simulink model "DC_motor"  (R2022b)
settings: Solver=VariableStepAuto  StartTime=0.0  StopTime=0.2  RelTol=1e-3
values from neighbouring files (symbols this model uses):
  b = 5.8/6*1e-4    (= 9.66666666667e-05)    [DC_motor_mfile.m]
  D_adm = 2*zeta_adm*wn_adm*M_adm    (= 20)    [DC_motor_mfile.m]    (also in oneDim_mfile.m = 1)
  g = 9.807    [DC_motor_mfile.m]    (also in oneDim_mfile.m)
  J = 5.8e-7    (= 5.8e-07)    [DC_motor_mfile.m]
  K_adm = wn_adm^2*M_adm    (= 100)    [DC_motor_mfile.m]    (also in oneDim_mfile.m = 2.5)
  K_D_pos = (2*zeta_m_pos*wn_m_pos*T - 1)/K    (= 0.0265230129141)    [DC_motor_mfile.m]
  K_D_pos_pass = 2*zeta_m_pos*wn_m_pos    (= 200)    [DC_motor_mfile.m]
  K_I_pos = 0    [DC_motor_mfile.m]
  K_P_pos = wn_m_pos^2 * T/K    (= 9.86111111111)    [DC_motor_mfile.m]
  K_P_pos_pass = wn_m_pos^2    (= 10000)    [DC_motor_mfile.m]
  Kb = 2.73e-3*(60/(2*pi))    (= 0.0260695796785)    [DC_motor_mfile.m]
  Km = 26.1e-3    (= 0.0261)    [DC_motor_mfile.m]
  L = 1    [DC_motor_mfile.m]
  m = 1    [DC_motor_mfile.m]    (also in oneDim_mfile.m = 0.5)
  M_adm = 1    [DC_motor_mfile.m]    (also in oneDim_mfile.m = 0.1)
  Ra = 7.1    [DC_motor_mfile.m]
  simpDC_gain = Km/(Ra*b+Kb*Km)    (= 19.0964054623)    [DC_motor_mfile.m]
  simpDC_timeconst = (Ra*J/(Ra*b+Kb*Km))    (= 0.00301298841738)    [DC_motor_mfile.m]
libraries: lib_robot x20
settings Model: Creator=chris  LastModifiedBy=chris

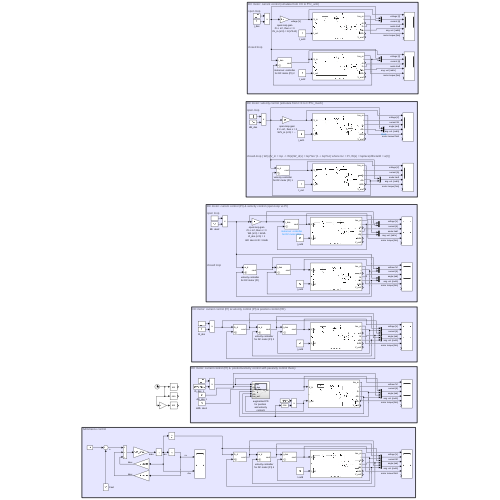
[thumbnail: Simulink's stored preview of the top-level diagram]
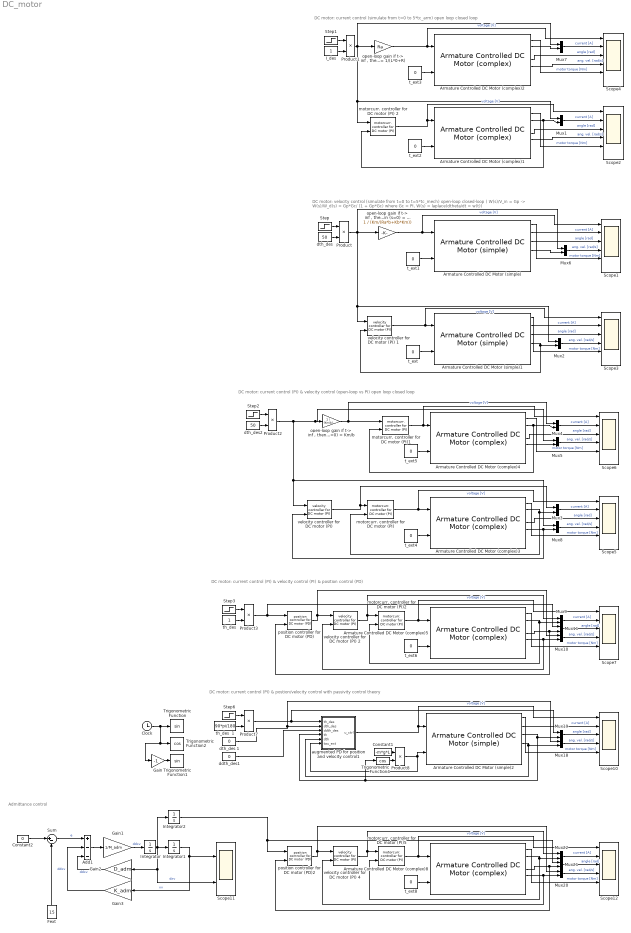
== system DC_motor ==
  note: Admittance control
  note: DC motor: current control (PI) & velocity control (PI) & position control (PD)
  note: DC motor: current control (PI) & velocity control (open-loop vs PI)
      |
      | open loop
      |
      |
      |
      |
      |
      |
      |
      |
      |
      |
      |
      |
      |
      |
      |
      | closed loop
  note: DC motor: current control (simulate from t=0 to 5*tc_arm)
      |
      | open loop
      |
      |
      |
      |
      |
      |
      |
      |
      |
      |
      | closed loop
  note: DC motor: velocity control (simulate from t=0 to t=5*tc_mech)
      |
      | open-loop
      |
      |
      |
      |
      |
      |
      |
      |
      |
      |
      |
      |
      |
      | closed-loop ( W(s)/V_in = Gp -> W(s)/W_d(s) = Gp*Gc/ (1 + Gp*Gc) where Gc = PI, W(s) = laplace(dtheta/dt = w(t))
  note: DC motor: current control (PI) & postion/velocity control with passivity control theory
  Add1 : Sum  Inputs=+--
  Armature Controlled DC Motor (complex){1..5,8} (6 alike) : lib_robot/Armature Controlled DC Motor (complex)  SystemSampleTime=-1  VariantActivationTime=update diagram  Latency=0  AutoFrameSizeCalculation=off
  Armature Controlled DC Motor (simple) : lib_robot/Armature Controlled DC Motor (simple)  SystemSampleTime=-1  VariantActivationTime=update diagram  Latency=0  AutoFrameSizeCalculation=off
  Armature Controlled DC Motor (simple)1 : lib_robot/Armature Controlled DC Motor (simple)  SystemSampleTime=-1  VariantActivationTime=update diagram  Latency=0  AutoFrameSizeCalculation=off
  Armature Controlled DC Motor (simple)2 : lib_robot/Armature Controlled DC Motor (simple)  SystemSampleTime=-1  VariantActivationTime=update diagram  Latency=0  AutoFrameSizeCalculation=off
  Clock : Clock
  Constant1 : Constant  Value=-m*g*L
  Constant2 : Constant  Value=0
  Fext : Constant  Value=15
  Gain : Gain  Gain=-1
  Gain1 : Gain  Gain=1/M_adm
  Gain2 : Gain  Gain=D_adm
  Gain3 : Gain  Gain=K_adm
  I_des : Constant
  Integrator : Integrator
  Integrator1 : Integrator
  Integrator2 : Integrator
  Mux{1..11,18..22} (16 alike) : Mux  Inputs=2
  Product{,1..3,7..8} (6 alike) : Product
  Scope{1..7,10,12} (9 alike) : Scope  NumInputPorts=6
  Scope11 : Scope  NumInputPorts=2
  Step{,1..3} (4 alike) : Step  Time=0  SampleTime=0
  Step6 : Step  Time=0.1  SampleTime=0
  Sum : Sum  Inputs=|+-
  Trigonometric Function : Trigonometry
  Trigonometric Function1 : Trigonometry
  Trigonometric Function2 : Trigonometry  Operator=cos
  Trigonometric Function4 : Trigonometry  Operator=cos
  augmented PD for position and velocity control1 : Subsystem
  ddth_des1 : Constant  Value=0
  dth_des : Constant  Value=50
  dth_des 1 : Constant  Value=0
  dth_des2 : Constant  Value=50
  motorcurr. controller for DC motor (PI){,1..2,5} (4 alike) : lib_robot/motorcurr. controller for DC motor (PI)  mask_K_P=K_P_cur  mask_K_I=K_I_cur
  motorcurr. controller for DC motor (PI) 2 : lib_robot/motorcurr. controller for DC motor (PI)  mask_K_P=K_P_cur  mask_K_I=K_I_cur
  "open-loop gain if t-> inf , then s = 0 I/V_in (s=0) = 1/(L*0+R)" : Gain  Gain=Ra
  "open-loop gain if t-> inf , then s = 0 W/I (s=0) = Km/b I/I_des (s=0) = 1 W/I_des (s=0) = Km/b" : Gain  Gain=1 / (Km/b)
  "open-loop gain if t-> inf , then s = 0 W/V_in (s=0) = ... " : Gain  Gain=1 / (Km/(Ra*b+Kb*Km))
  position controller for DC motor (PD) : lib_robot/position controller for DC motor (PD)  P=K_P_pos  I=K_I_pos  D=K_D_pos  N=100
  position controller for DC motor (PD)2 : lib_robot/position controller for DC motor (PD)  P=K_P_pos  I=K_I_pos  D=K_D_pos  N=100
  t_ext{,1..6,8} (8 alike) : Constant  Value=0
  th_des : Constant
  th_des  1 : Constant  Value=90*pi/180
  velocity controller for DC motor (PI) {,1..2,4} (4 alike) : lib_robot/velocity controller for DC motor (PI)  mask_K_P=K_P_vel  mask_K_I=K_I_vel
  wires:
  t_ext/1 -> Armature Controlled DC Motor (simple)1/2
  Product/1 -> "open-loop gain if t-> inf , then s = 0 W/V_in (s=0) = ... "/1, Mux6/1, velocity controller for DC motor (PI) 1/1, Mux2/1
  Armature Controlled DC Motor (simple)1/3 -> Scope3/3  "angle [rad]"
  Armature Controlled DC Motor (simple)1/4 -> velocity controller for DC motor (PI) 1/2, Mux2/2
  velocity controller for DC motor (PI) 1/1 -> Scope3/1, Armature Controlled DC Motor (simple)1/1  "voltage [V]"
  Armature Controlled DC Motor (simple)1/2 -> Scope3/2  "current [A]"
  Mux2/1 -> Scope3/4  "ang. vel. [rad/s]"
  Armature Controlled DC Motor (simple)1/1 -> Scope3/5  "motor torque [Nm]"
  t_ext1/1 -> Armature Controlled DC Motor (simple)/2
  Armature Controlled DC Motor (simple)/3 -> Scope1/3  "angle [rad]"
  Armature Controlled DC Motor (simple)/1 -> Scope1/5  "motor torque [Nm]"
  Mux6/1 -> Scope1/4  "ang. vel. [rad/s]"
  "open-loop gain if t-> inf , then s = 0 W/V_in (s=0) = ... "/1 -> Scope1/1, Armature Controlled DC Motor (simple)/1  "voltage [V]"
  Armature Controlled DC Motor (simple)/2 -> Scope1/2  "current [A]"
  Step/1 -> Product/1
  dth_des/1 -> Product/2
  Armature Controlled DC Motor (complex)1/4 -> Scope2/3  "angle [rad]"
  Armature Controlled DC Motor (complex)1/1 -> Scope2/5  "motor torque [Nm]"
  Armature Controlled DC Motor (complex)1/2 -> motorcurr. controller for DC motor (PI) 2/2, Mux1/2
  t_ext2/1 -> Armature Controlled DC Motor (complex)1/2
  Product1/1 -> "open-loop gain if t-> inf , then s = 0 I/V_in (s=0) = 1/(L*0+R)"/1, Mux7/1, motorcurr. controller for DC motor (PI) 2/1, Mux1/1
  Armature Controlled DC Motor (complex)1/5 -> Scope2/4  "ang. vel. [rad/s]"
  motorcurr. controller for DC motor (PI) 2/1 -> Scope2/1, Armature Controlled DC Motor (complex)1/1  "voltage [V]"
  Mux1/1 -> Scope2/2  "current [A]"
  t_ext3/1 -> Armature Controlled DC Motor (complex)2/2
  Armature Controlled DC Motor (complex)2/1 -> Scope4/5  "motor torque [Nm]"
  Mux7/1 -> Scope4/2  "current [A]"
  Armature Controlled DC Motor (complex)2/4 -> Scope4/3  "angle [rad]"
  "open-loop gain if t-> inf , then s = 0 I/V_in (s=0) = 1/(L*0+R)"/1 -> Scope4/1, Armature Controlled DC Motor (complex)2/1  "voltage [V]"
  Armature Controlled DC Motor (complex)2/5 -> Scope4/4  "ang. vel. [rad/s]"
  t_ext4/1 -> Armature Controlled DC Motor (complex)3/2
  Armature Controlled DC Motor (complex)3/5 -> "velocity controller for DC motor (PI) "/2, Mux8/2
  Product2/1 -> "velocity controller for DC motor (PI) "/1, Mux8/1, Mux5/1, "open-loop gain if t-> inf , then s = 0 W/I (s=0) = Km/b I/I_des (s=0) = 1 W/I_des (s=0) = Km/b"/1
  t_ext5/1 -> Armature Controlled DC Motor (complex)4/2
  Mux5/1 -> Scope6/4  "ang. vel. [rad/s]"
  Armature Controlled DC Motor (complex)4/1 -> Scope6/5  "motor torque [Nm]"
  motorcurr. controller for DC motor (PI)1/1 -> Scope6/1, Armature Controlled DC Motor (complex)4/1  "voltage [V]"
  Armature Controlled DC Motor (complex)4/4 -> Scope6/3  "angle [rad]"
  Mux4/1 -> Scope6/2  "current [A]"
  Armature Controlled DC Motor (complex)4/2 -> motorcurr. controller for DC motor (PI)1/2, Mux4/2
  "open-loop gain if t-> inf , then s = 0 W/I (s=0) = Km/b I/I_des (s=0) = 1 W/I_des (s=0) = Km/b"/1 -> motorcurr. controller for DC motor (PI)1/1, Mux4/1
  Armature Controlled DC Motor (simple)/4 -> Mux6/2
  Armature Controlled DC Motor (complex)2/2 -> Mux7/2
  Armature Controlled DC Motor (complex)4/5 -> Mux5/2
  Mux3/1 -> Scope5/2  "current [A]"
  Mux8/1 -> Scope5/4  "ang. vel. [rad/s]"
  Armature Controlled DC Motor (complex)3/2 -> motorcurr. controller for DC motor (PI)/2, Mux3/2
  Armature Controlled DC Motor (complex)3/4 -> Scope5/3  "angle [rad]"
  Armature Controlled DC Motor (complex)3/1 -> Scope5/5  "motor torque [Nm]"
  "velocity controller for DC motor (PI) "/1 -> motorcurr. controller for DC motor (PI)/1, Mux3/1
  motorcurr. controller for DC motor (PI)/1 -> Armature Controlled DC Motor (complex)3/1, Scope5/1  "voltage [V]"
  I_des/1 -> Product1/2
  Step1/1 -> Product1/1
  Step2/1 -> Product2/1
  dth_des2/1 -> Product2/2
  Mux10/1 -> Scope7/4  "ang. vel. [rad/s]"
  Armature Controlled DC Motor (complex)5/1 -> Scope7/5  "motor torque [Nm]"
  velocity controller for DC motor (PI) 2/1 -> motorcurr. controller for DC motor (PI)2/1, Mux9/1
  t_ext6/1 -> Armature Controlled DC Motor (complex)5/2
  Armature Controlled DC Motor (complex)5/5 -> velocity controller for DC motor (PI) 2/2, Mux10/2
  Mux9/1 -> Scope7/2  "current [A]"
  motorcurr. controller for DC motor (PI)2/1 -> Armature Controlled DC Motor (complex)5/1, Scope7/1  "voltage [V]"
  Armature Controlled DC Motor (complex)5/4 -> Mux11/2, position controller for DC motor (PD)/2
  Armature Controlled DC Motor (complex)5/2 -> Mux9/2, motorcurr. controller for DC motor (PI)2/2
  Step3/1 -> Product3/1
  th_des/1 -> Product3/2
  Product3/1 -> Mux11/1, position controller for DC motor (PD)/1
  position controller for DC motor (PD)/1 -> Mux10/1, velocity controller for DC motor (PI) 2/1
  Mux11/1 -> Scope7/3  "angle [rad]"
  Clock/1 -> Gain/1, Trigonometric Function2/1, Trigonometric Function/1
  Gain/1 -> Trigonometric Function1/1
  Mux18/1 -> Scope10/4  "ang. vel. [rad/s]"
  Armature Controlled DC Motor (simple)2/2 -> Scope10/2  "current [A]"
  Constant1/1 -> Product8/1
  Step6/1 -> Product7/1
  augmented PD for position and velocity control1/1(u_ctrl) -> Scope10/1, Armature Controlled DC Motor (simple)2/1  "voltage [V]"
  ddth_des1/1 -> augmented PD for position and velocity control1/3(ddth_des)
  dth_des 1/1 -> augmented PD for position and velocity control1/2(dth_des), Mux18/1
  th_des  1/1 -> Product7/2
  Product7/1 -> Mux19/1, augmented PD for position and velocity control1/1(th_des)
  Trigonometric Function4/1 -> Product8/2
  Armature Controlled DC Motor (simple)2/1 -> Scope10/5  "motor torque [Nm]"
  Product8/1 -> augmented PD for position and velocity control1/6(tau_ext), Armature Controlled DC Motor (simple)2/2
  Armature Controlled DC Motor (simple)2/4 -> augmented PD for position and velocity control1/5(dth), Mux18/2
  Armature Controlled DC Motor (simple)2/3 -> Trigonometric Function4/1, augmented PD for position and velocity control1/4(th), Mux19/2
  Mux19/1 -> Scope10/3  "angle [rad]"
  Integrator1/1 -> Scope11/1, Gain3/1  "xv"
  Integrator/1 -> Integrator2/1, Scope11/2, Gain2/1, Integrator1/1  "dxv"
  Add1/1 -> Gain1/1
  Gain1/1 -> Integrator/1  "ddxv"
  Gain2/1 -> Add1/3  "ddxv"
  Gain3/1 -> Add1/2  "ddxv"
  Armature Controlled DC Motor (complex)8/1 -> Scope12/5  "motor torque [Nm]"
  t_ext8/1 -> Armature Controlled DC Motor (complex)8/2
  Armature Controlled DC Motor (complex)8/2 -> Mux22/2, motorcurr. controller for DC motor (PI)5/2
  Mux20/1 -> Scope12/4  "ang. vel. [rad/s]"
  position controller for DC motor (PD)2/1 -> Mux20/1, velocity controller for DC motor (PI) 4/1
  Mux22/1 -> Scope12/2  "current [A]"
  velocity controller for DC motor (PI) 4/1 -> motorcurr. controller for DC motor (PI)5/1, Mux22/1
  Integrator2/1 -> position controller for DC motor (PD)2/1, Mux21/1
  Armature Controlled DC Motor (complex)8/5 -> velocity controller for DC motor (PI) 4/2, Mux20/2
  motorcurr. controller for DC motor (PI)5/1 -> Armature Controlled DC Motor (complex)8/1, Scope12/1  "voltage [V]"
  Armature Controlled DC Motor (complex)8/4 -> Mux21/2, position controller for DC motor (PD)2/2
  Mux21/1 -> Scope12/3  "angle [rad]"
  Fext/1 -> Sum/2
  Sum/1 -> Add1/1  "e"
  Constant2/1 -> Sum/1

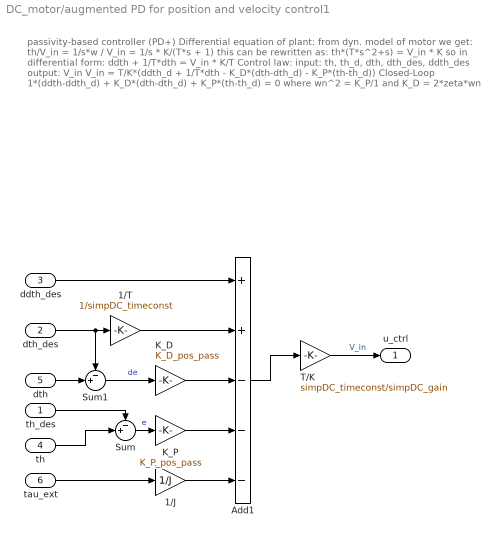
== system DC_motor/augmented PD for position and velocity control1 ==
  note: passivity-based controller (PD+)
      |
      | Differential equation of plant:
      |   from dyn. model of motor we get:  th/V_in = 1/s*w / V_in = 1/s * K/(T*s + 1)
      |   this can be rewritten as:                 th*(T*s^2+s) = V_in * K
      |   so in differential form:                     ddth + 1/T*dth = V_in * K/T
      |
      | Control law:
      |   input:   th, th_d, dth, dth_des, ddth_des
      |   output: V_in
      |   V_in = T/K*(ddth_d + 1/T*dth - K_D*(dth-dth_d) - K_P*(th-th_d))
      |
      | Closed-Loop
      |    1*(ddth-ddth_d) + K_D*(dth-dth_d) + K_P*(th-th_d) = 0
      |    where   wn^2 = K_P/1     and       K_D = 2*zeta*wn
  th_des : Inport
  dth_des : Inport  Port=2
  ddth_des : Inport  Port=3
  th : Inport  Port=4
  dth : Inport  Port=5
  tau_ext : Inport  Port=6
  1/J : Gain  Gain=1/J
  1/T : Gain  Gain=1/simpDC_timeconst
  Add1 : Sum  Inputs=++---
  K_D : Gain  Gain=K_D_pos_pass
  K_P : Gain  Gain=K_P_pos_pass
  Sum : Sum  Inputs=-+|
  Sum1 : Sum  Inputs=-+|
  T/K : Gain  Gain=simpDC_timeconst/simpDC_gain
  u_ctrl : Outport
  wires:
  ddth_des/1 -> Add1/1
  T/K/1 -> u_ctrl/1  "V_in"
  Add1/1 -> T/K/1
  th_des/1 -> Sum/1
  Sum/1 -> K_P/1  "e"
  Sum1/1 -> K_D/1  "de"
  dth_des/1 -> Sum1/1, 1/T/1
  1/T/1 -> Add1/2
  dth/1 -> Sum1/2
  K_D/1 -> Add1/3
  th/1 -> Sum/2
  K_P/1 -> Add1/4
  1/J/1 -> Add1/5
  tau_ext/1 -> 1/J/1
